simulink model "rct_diesel"  (R2022a)
settings: Solver=FixedStepDiscrete  StartTime=0.0  StopTime=140  RelTol=1e-3
PreLoadFcn:
  | %% Plant model
  | load DieselEngine Plant
  | [a,b,c,d] = ssdata(Plant);
  | 
  | %% Bias computation for simulation
  | % Fuel  mass and engine speed at operating point
  | D0 = [12;2100];
  | 
  | % Nominal VGT and EGR positions at operating point
  | U0 = [0.375;2.5];
  | 
  | % Corresponding steady-state values of BOOST and EGR
  | X0 = (eye(4)-a)\(b*[U0;D0]);
  | Y0 = c*X0+d*[U0;D0];
  | 
  | % Choose State Space Controller as default variant
  | MODE = 1;
undefined symbols (not defined in the file or in its folder): DiscIntNeverNeededParam, Plant, sigbuilder_block
settings Model: Creator=The MathWorks, Inc.  LastModifiedBy=The MathWorks, Inc.
settings SolverCC: AlgebraicLoopSolver=TrustRegion  MaxZcPerStep=1
settings DataIOCC: LimitDataPoints=on  SaveFormat=Array  ReturnWorkspaceOutputs=off
settings OptimizationCC: ExpressionDepthLimit=2147483647  LifeSpan=inf
settings DebuggingCC: UnderspecifiedInitializationDetection=Classic  MergeDetectMultiDrivingBlocksExec=none  SolverPrmCheckMsg=warning  UnconnectedInputMsg=warning  UnconnectedOutputMsg=warning  UnconnectedLineMsg=warning  StateNameClashWarn=warning  SFUnexpectedBacktrackingDiag=warning  SFNoUnconditionalDefaultTransitionDiag=warning  SFExecutionAtInitializationDiag=none  SFMachineParentedDataDiag=warning  ArithmeticOperatorsInVariantConditions=warning
settings HardwareCC: ProdBitPerPointer=32  ProdBitPerSizeT=32  ProdBitPerPtrDiffT=32  ProdLargestAtomicFloat=None  ProdIntDivRoundTo=Undefined  ProdEndianess=Unspecified  ProdWordSize=32  ProdHWDeviceType=32-bit Generic
settings ModelReferenceCC: PropagateSignalLabelsOutOfModel=off
settings SFSimCC: SimUseLocalCustomCode=off  CustomCodeUndefinedFunction=UseInterfaceOnly
settings RTWCC: RTWUseLocalCustomCode=off  DLArmComputeVersion=19.05
settings CodeAppCC: StateflowObjectComments=on
settings GRTTargetCC: TargetLangStandard=C89/C90 (ANSI)
settings ConfigComp: CovMetricSettings=dw  CovSaveCumulativeToWorkspaceVar=on  CovSaveSingleToWorkspaceVar=on  CovExternalEMLEnable=off  CovSFcnEnable=off

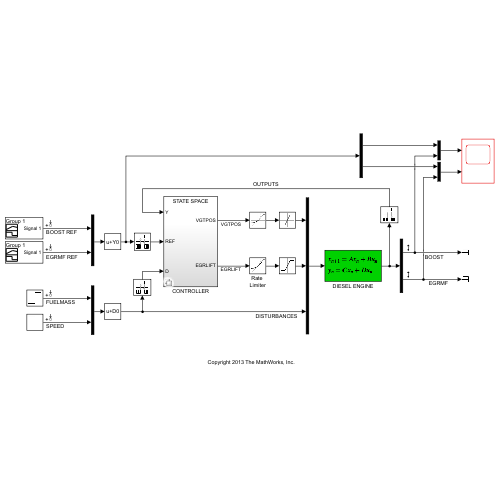
[thumbnail: Simulink's stored preview of the top-level diagram]
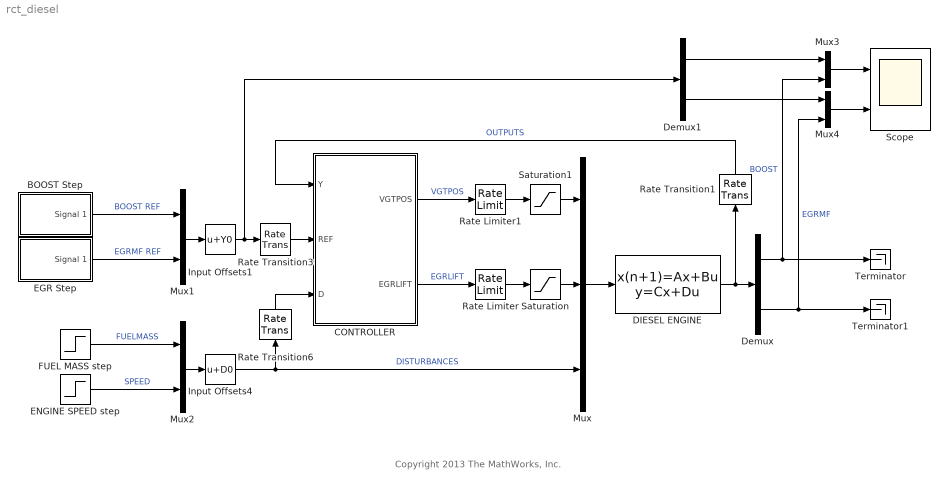
== system rct_diesel ==
  note: Copyright 2013 The MathWorks, Inc.
  BOOST Step : Subsystem  Tag=STV Subsys  LoadFcn=sigbuilder_block('load');  StartFcn=sigbuilder_block('start');  StopFcn=sigbuilder_block('stop');  ClipboardFcn=sigbuilder_block('clipboard');  mask(Sigbuilder block){tuvar=[0:10]}
      mask help: Simulink:masks:SigbuilderBlock_MD
      mask init:
      | if ~strcmp(get_param(bdroot(gcbh),'SimulationStatus'),'stopped') tuvar = sigbuilder_block('maskInit'); end
      settings: CopyFcn=sigbuilder_block('copy');  DeleteFcn=sigbuilder_block('delete');  ModelCloseFcn=sigbuilder_block('modelClose');  PreSaveFcn=sigbuilder_block('preSave');  PauseFcn=sigbuilder_block('pause');  ContinueFcn=sigbuilder_block('continue');  NameChangeFcn=sigbuilder_block('namechange');  OpenFcn=sigbuilder_block('open',[315 191.25 550.5 395.25 ]);  CloseFcn=sigbuilder_block('close');
      mask Display: plot(0, 0, 100, 100,[2, 2, 32, 32, 2], [68, 8, 8, 68, 68],[32, 2], [38, 38], [32, 19, 2],[53, 60, 44], [32, 17, 17, 2],[16, 16, 31, 31]);txt = getActiveGroup(gcbh);text(2, 100, txt,'verticalAlignment', 'top');
  CONTROLLER : Subsystem  Variant=on
  DIESEL ENGINE : DiscreteStateSpace  A=Plant.a  B=Plant.b  C=Plant.c  D=Plant.d  InitialCondition=X0  SampleTime=Plant.Ts
  Demux : Demux  Outputs=2
  Demux1 : Demux  Outputs=2
  EGR Step : Subsystem  Tag=STV Subsys  LoadFcn=sigbuilder_block('load');  StartFcn=sigbuilder_block('start');  StopFcn=sigbuilder_block('stop');  ClipboardFcn=sigbuilder_block('clipboard');  mask(Sigbuilder block){tuvar=[0:10]}
      mask help: Simulink:masks:SigbuilderBlock_MD
      mask init:
      | if ~strcmp(get_param(bdroot(gcbh),'SimulationStatus'),'stopped') tuvar = sigbuilder_block('maskInit'); end
      settings: CopyFcn=sigbuilder_block('copy');  DeleteFcn=sigbuilder_block('delete');  ModelCloseFcn=sigbuilder_block('modelClose');  PreSaveFcn=sigbuilder_block('preSave');  PauseFcn=sigbuilder_block('pause');  ContinueFcn=sigbuilder_block('continue');  NameChangeFcn=sigbuilder_block('namechange');  OpenFcn=sigbuilder_block('open',[403.5 199.5 550.5 395.25 ]);  CloseFcn=sigbuilder_block('close');
      mask Display: plot(0, 0, 100, 100,[2, 2, 32, 32, 2], [68, 8, 8, 68, 68],[32, 2], [38, 38], [32, 19, 2],[53, 60, 44], [32, 17, 17, 2],[16, 16, 31, 31]);txt = getActiveGroup(gcbh);text(2, 100, txt,'verticalAlignment', 'top');
  ENGINE SPEED step : Step  Time=110  After=-200  SampleTime=0
  FUEL MASS step : Step  Time=90  After=5  SampleTime=0
  Input Offsets1 : Bias  Bias=Y0  SaturateOnIntegerOverflow=off
  Input Offsets4 : Bias  Bias=D0  SaturateOnIntegerOverflow=off
  Mux : Mux  Inputs=3
  Mux{1..4} (4 alike) : Mux  Inputs=2
  Rate Limiter : RateLimiter  RisingSlewLimit=5  FallingSlewLimit=-5  SampleTimeMode=inherited  InitialCondition=-1
  Rate Limiter1 : RateLimiter  RisingSlewLimit=0.9  FallingSlewLimit=-0.9  SampleTimeMode=inherited
  Rate Transition1 : RateTransition  OutPortSampleTime=0.2
  Rate Transition3 : RateTransition  OutPortSampleTime=0.2
  Rate Transition6 : RateTransition  OutPortSampleTime=0.2
  Saturation : Saturate  UpperLimit=5  LowerLimit=0
  Saturation1 : Saturate  UpperLimit=1  LowerLimit=0
  Scope : Scope  NumInputPorts=2
  Terminator : Terminator
  Terminator1 : Terminator
  wires:
  DIESEL ENGINE/1 -> Demux/1, Rate Transition1/1
  BOOST Step/1(Signal 1) -> Mux1/1  "BOOST REF"
  EGR Step/1(Signal 1) -> Mux1/2  "EGRMF REF"
  ENGINE SPEED step/1 -> Mux2/2  "SPEED"
  FUEL MASS step/1 -> Mux2/1  "FUELMASS"
  Rate Limiter/1 -> Saturation/1
  Rate Limiter1/1 -> Saturation1/1
  Saturation/1 -> Mux/2
  Saturation1/1 -> Mux/1
  Demux/2 -> Terminator1/1, Mux4/2  "EGRMF"
  Input Offsets1/1 -> Demux1/1, Rate Transition3/1
  Mux1/1 -> Input Offsets1/1
  Mux2/1 -> Input Offsets4/1
  Input Offsets4/1 -> Rate Transition6/1, Mux/3  "DISTURBANCES"
  Demux/1 -> Terminator/1, Mux3/2  "BOOST"
  Rate Transition1/1 -> CONTROLLER/1(Y)  "OUTPUTS"
  Rate Transition3/1 -> CONTROLLER/2(REF)
  Mux/1 -> DIESEL ENGINE/1
  Rate Transition6/1 -> CONTROLLER/3(D)
  Mux3/1 -> Scope/1
  Mux4/1 -> Scope/2
  Demux1/1 -> Mux3/1
  Demux1/2 -> Mux4/1
  CONTROLLER/1(VGTPOS) -> Rate Limiter1/1  "VGTPOS"
  CONTROLLER/2(EGRLIFT) -> Rate Limiter/1  "EGRLIFT"

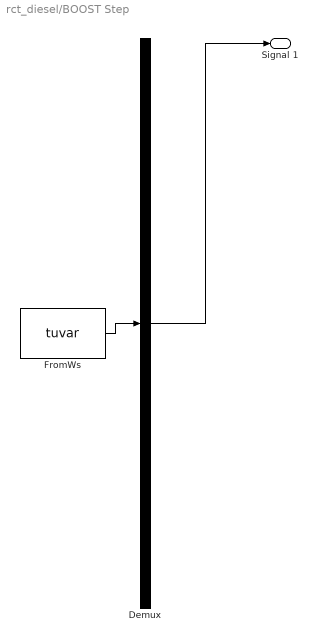
== system rct_diesel/BOOST Step ==
  Demux : Demux  Tag=STV Demux  Outputs=1
      settings: DisplayOption=none
  FromWs : FromWorkspace  Tag=STV FromWs  VariableName=tuvar
      SigBuilderData=|
      | common.afterFinalStr = 'Extrapolate'
      | common.sampleTime = 0
      | dataSet.timeRange = [0 40]
      | dataSet.name = 'Group 1'
      | sbobj.Groups.Name = 'Group 1'
      | sbobj.Groups.Signals.Name = 'Signal 1'
      | sbobj.Groups.Signals.XData = [0 15.1 15.1 30 30 40]
      | sbobj.Groups.Signals.YData = [0 0 10 10 0 0]
      | sbobj.Groups.TimeRange = [0 40]
  Signal 1 : Outport  Tag=STV Outport  VectorParamsAs1DForOutWhenUnconnected=off
  wires:
  Demux/1 -> Signal 1/1
  FromWs/1 -> Demux/1

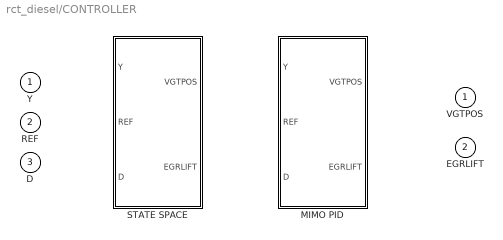
== system rct_diesel/CONTROLLER ==
  Y : Inport
  REF : Inport  Port=2
  D : Inport  Port=3
  MIMO PID : Subsystem  VariantControl=MODE==2
  STATE SPACE : Subsystem  VariantControl=MODE==1
  VGTPOS : Outport  VectorParamsAs1DForOutWhenUnconnected=off
  EGRLIFT : Outport  Port=2  VectorParamsAs1DForOutWhenUnconnected=off

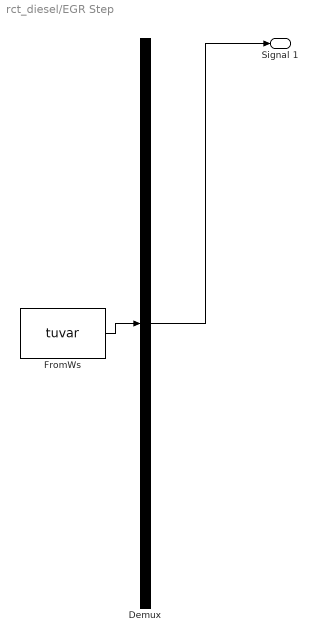
== system rct_diesel/EGR Step ==
  Demux : Demux  Tag=STV Demux  Outputs=1
      settings: DisplayOption=none
  FromWs : FromWorkspace  Tag=STV FromWs  VariableName=tuvar
      SigBuilderData=|
      | common.afterFinalStr = 'Extrapolate'
      | common.sampleTime = 0
      | dataSet.timeRange = [0 100]
      | dataSet.name = 'Group 1'
      | sbobj.Groups.Name = 'Group 1'
      | sbobj.Groups.Signals.Name = 'Signal 1'
      | sbobj.Groups.Signals.XData = [0 50 50 70 70 100]
      | sbobj.Groups.Signals.YData = [0 0 3 3 0 0]
      | sbobj.Groups.TimeRange = [0 100]
  Signal 1 : Outport  Tag=STV Outport  VectorParamsAs1DForOutWhenUnconnected=off
  wires:
  FromWs/1 -> Demux/1
  Demux/1 -> Signal 1/1

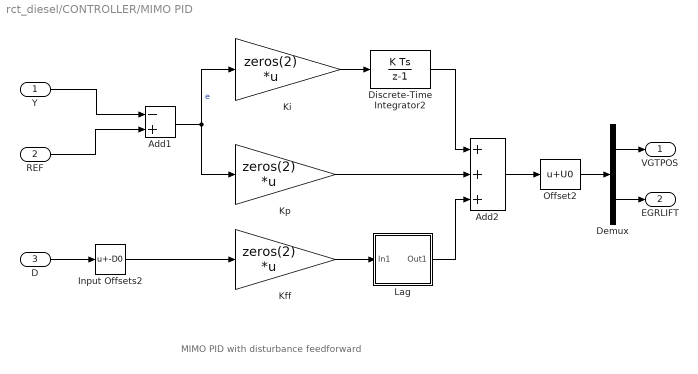
== system rct_diesel/CONTROLLER/MIMO PID ==
  note: MIMO PID with disturbance feedforward
  Y : Inport
  REF : Inport  Port=2
  D : Inport  Port=3
  Add1 : Sum  Inputs=-+
  Add2 : Sum  Inputs=+++
  Demux : Demux  Outputs=2
  Discrete-Time Integrator2 : DiscreteIntegrator  SampleTime=0.2  ICPrevOutput=DiscIntNeverNeededParam  ICPrevScaledInput=DiscIntNeverNeededParam
  Input Offsets2 : Bias  Bias=-D0  SaturateOnIntegerOverflow=off
  Kff : Gain  Gain=zeros(2)  Multiplication=Matrix(K*u)
  Ki : Gain  Gain=zeros(2)  Multiplication=Matrix(K*u)
  Kp : Gain  Gain=zeros(2)  Multiplication=Matrix(K*u)
  Lag : Subsystem
  Offset2 : Bias  Bias=U0  SaturateOnIntegerOverflow=off
  VGTPOS : Outport  VectorParamsAs1DForOutWhenUnconnected=off
  EGRLIFT : Outport  Port=2  VectorParamsAs1DForOutWhenUnconnected=off
  wires:
  REF/1 -> Add1/2
  Y/1 -> Add1/1
  Discrete-Time Integrator2/1 -> Add2/1
  Demux/2 -> EGRLIFT/1
  Offset2/1 -> Demux/1
  Kff/1 -> Lag/1(In1)
  Kp/1 -> Add2/2
  Ki/1 -> Discrete-Time Integrator2/1
  Input Offsets2/1 -> Kff/1
  Add2/1 -> Offset2/1
  D/1 -> Input Offsets2/1
  Add1/1 -> Ki/1, Kp/1  "e"
  Demux/1 -> VGTPOS/1
  Lag/1(Out1) -> Add2/3

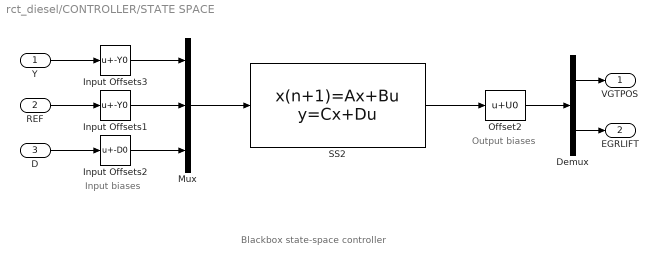
== system rct_diesel/CONTROLLER/STATE SPACE ==
  note: Blackbox state-space controller
  note: Input biases
  note: Output biases
  Y : Inport
  REF : Inport  Port=2
  D : Inport  Port=3
  Demux : Demux  Outputs=2
  Input Offsets1 : Bias  Bias=-Y0  SaturateOnIntegerOverflow=off
  Input Offsets2 : Bias  Bias=-D0  SaturateOnIntegerOverflow=off
  Input Offsets3 : Bias  Bias=-Y0  SaturateOnIntegerOverflow=off
  Mux : Mux  Inputs=3
  Offset2 : Bias  Bias=U0  SaturateOnIntegerOverflow=off
  SS2 : DiscreteStateSpace  A=0.9*eye(2)  B=ones(2,6)  C=zeros(2,2)  D=zeros(2,6)  SampleTime=0.2
  VGTPOS : Outport  VectorParamsAs1DForOutWhenUnconnected=off
  EGRLIFT : Outport  Port=2  VectorParamsAs1DForOutWhenUnconnected=off
  wires:
  Demux/1 -> VGTPOS/1
  D/1 -> Input Offsets2/1
  Offset2/1 -> Demux/1
  Demux/2 -> EGRLIFT/1
  SS2/1 -> Offset2/1
  Mux/1 -> SS2/1
  REF/1 -> Input Offsets1/1
  Input Offsets2/1 -> Mux/3
  Input Offsets1/1 -> Mux/2
  Y/1 -> Input Offsets3/1
  Input Offsets3/1 -> Mux/1

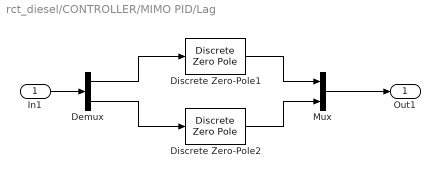
== system rct_diesel/CONTROLLER/MIMO PID/Lag ==
  In1 : Inport
  Demux : Demux  Outputs=2
  Discrete Zero-Pole1 : DiscreteZeroPole  Zeros=0.9975  Poles=0.9993  Gain=1  SampleTime=0.2
  Discrete Zero-Pole2 : DiscreteZeroPole  Zeros=0.9975  Poles=0.9993  Gain=1  SampleTime=0.2
  Mux : Mux  Inputs=2
  Out1 : Outport  VectorParamsAs1DForOutWhenUnconnected=off
  wires:
  In1/1 -> Demux/1
  Demux/1 -> Discrete Zero-Pole1/1
  Demux/2 -> Discrete Zero-Pole2/1
  Discrete Zero-Pole1/1 -> Mux/1
  Discrete Zero-Pole2/1 -> Mux/2
  Mux/1 -> Out1/1
